simulink model "generic"  (Simulink 10.3)
settings: Solver=ode45  StartTime=0.0  StopTime=inf  RelTol=1e-3  EnableMultiTasking=on
libraries: CarMaker4SL x62, simulink x6
(part 3 of 3)

== system generic/CarMaker/VehicleControl/CreateBus VhclCtrl/Braking/Subsystem6/While Iterator Subsystem/If Action Subsystem1/If Action Subsystem4 ==
  Action Port : ActionPort  ActionPortLabel=else
